simulink model "RuidoFiltrado"  (Simulink 7.5)
settings: Solver=ode3  StartTime=Intime  StopTime=Sttime  FixedStep=dt  RelTol=1e-3
values from neighbouring files (symbols this model uses):
  dt = 10^-3    (= 0.001)    [RuidoFiltroN.m]
  FTf = 1/mag*FTfp    [Filtros.m]    (also in RuidoFiltroN.m)
  gain = 0.01    [RuidoFiltroN.m]
  Intime = 0    [Filtros.m]    (also in RuidoFiltroN.m)
  tsub = 2    [Filtros.m]    (also in RuidoFiltroN.m)
libraries: simulink x1
settings Model: Creator=FVOliveira  LastModifiedBy=Ferdinando
settings DebuggingCC: StrictBusMsg=Warning

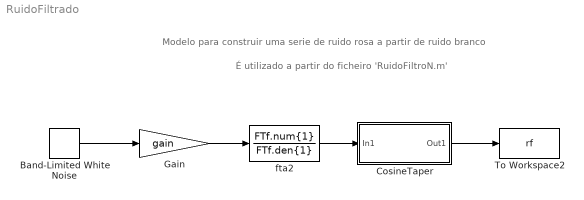
== system RuidoFiltrado ==
  note: Modelo para construir uma serie de ruido rosa a partir de ruido branco
  note: É utilizado a partir do ficheiro 'RuidoFiltroN.m'
  Band-Limited White Noise : simulink/Sources/Band-Limited White Noise  SystemSampleTime=-1  Cov=1  Ts=dt  seed=[23341]
  CosineTaper : Subsystem  TreatAsAtomicUnit=on
  Gain : Gain  Gain=gain  ParameterDataType=fixdt(1, 16)  ParameterScaling=2^0  OutDataType=fixdt(1, 16)  OutScaling=2^0
  To Workspace2 : ToWorkspace  VariableName=rf  SampleTime=-1  SaveFormat=Structure With Time
  fta2 : TransferFcn  Numerator=FTf.num{1}  Denominator=FTf.den{1}
  wires:
  Gain/1 -> fta2/1
  Band-Limited White Noise/1 -> Gain/1
  fta2/1 -> CosineTaper/1(In1)
  CosineTaper/1(Out1) -> To Workspace2/1

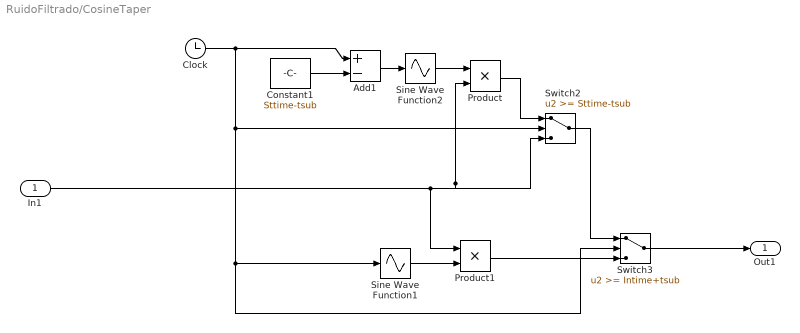
== system RuidoFiltrado/CosineTaper ==
  In1 : Inport  OutDataType=sfix(16)  OutScaling=2^0
  Add1 : Sum  Inputs=+-  OutDataType=sfix(16)  OutScaling=2^-10
  Clock : Clock
      settings: Decimation=10
  Constant1 : Constant  Value=Sttime-tsub  OutDataType=sfix(16)  OutScaling=2^0
  Product : Product  OutDataType=sfix(16)  OutScaling=2^0  RndMeth=Zero
  Product1 : Product  OutDataType=sfix(16)  OutScaling=2^0  RndMeth=Zero
  Sine Wave Function1 : Sin  TimeSource=Use external signal  Amplitude=0.5  Bias=0.5  Frequency=pi/tsub  Phase=-pi/2  Samples=10  SampleTime=0  Offset=0
  Sine Wave Function2 : Sin  TimeSource=Use external signal  Amplitude=0.5  Bias=0.5  Frequency=pi/tsub  Phase=pi/2  Samples=10  SampleTime=0  Offset=0
  Switch2 : Switch  Threshold=Sttime-tsub  OutDataType=fixdt(1, 16)  OutScaling=2^0
  Switch3 : Switch  Threshold=Intime+tsub  OutDataType=fixdt(1, 16)  OutScaling=2^0
  Out1 : Outport  OutDataType=sfix(16)  OutScaling=2^0
  wires:
  Constant1/1 -> Add1/2
  Add1/1 -> Sine Wave Function2/1
  Sine Wave Function2/1 -> Product/1
  Product/1 -> Switch2/1
  In1/1 -> Product/2, Switch2/3, Product1/1
  Switch2/1 -> Switch3/1
  Clock/1 -> Add1/1, Switch2/2, Sine Wave Function1/1, Switch3/2
  Sine Wave Function1/1 -> Product1/2
  Product1/1 -> Switch3/3
  Switch3/1 -> Out1/1
